simulink model "bomb"  (R2018b)
settings: Solver=FixedStepAuto  StartTime=0.0  StopTime=inf  FixedStep=0.01  RelTol=1e-3
values from neighbouring files (symbols this model uses):
  caliber = 0.299    [init.m]
  g = 9.8    [init.m]
  specified_drag_coefficient = 0.16    [init.m]
  standard_density = 1.225    [init.m]
  standard_drag_coefficient = 0.659    [init.m]
  standard_temperature = 288.4    [init.m]
  weight = 216.5    [init.m]
libraries: aerolibatmos2 x1, aerolibasang x1
settings Model: Creator=ysq  LastModifiedBy=ysq

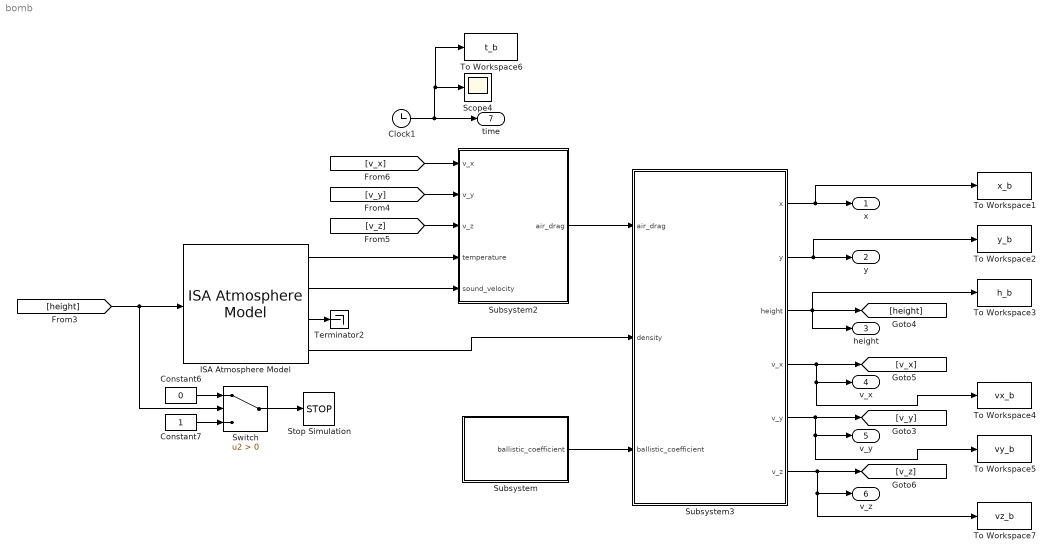
== system bomb ==
  Clock1 : Clock
  Constant6 : Constant  Value=0
  Constant7 : Constant
  ISA Atmosphere Model : aerolibatmos2/ISA Atmosphere Model  custom=off  g=9.80665  gamma=1.4  R=287.0531  L=0.0065  h_trop=11000  h_strat=20000  rho0=1.225  P0=101325  T0=288.15  h0=0
      settings: SourceProductName=Aerospace Blockset
  Scope4 : Scope
  Stop Simulation : Stop
  Subsystem : Subsystem
  Subsystem2 : Subsystem
  Subsystem3 : Subsystem
  Switch : Switch  Criteria=u2 > Threshold
  Terminator2 : Terminator
  To Workspace1 : ToWorkspace  VariableName=x_b  SampleTime=-1
  To Workspace2 : ToWorkspace  VariableName=y_b  SampleTime=-1
  To Workspace3 : ToWorkspace  VariableName=h_b  SampleTime=-1
  To Workspace4 : ToWorkspace  VariableName=vx_b  SampleTime=-1
  To Workspace5 : ToWorkspace  VariableName=vy_b  SampleTime=-1
  To Workspace6 : ToWorkspace  VariableName=t_b  SampleTime=-1
  To Workspace7 : ToWorkspace  VariableName=vz_b  SampleTime=-1
  x : Outport
  y : Outport  Port=2
  height : Outport  Port=3
  v_x : Outport  Port=4
  v_y : Outport  Port=5
  v_z : Outport  Port=6
  time : Outport  Port=7
  wires:
  Constant7/1 -> Switch/3
  [v_z] -> Subsystem2/3(v_z)
  [height] -> ISA Atmosphere Model/1, Switch/2
  Subsystem3/2(y) -> y/1, To Workspace2/1
  ISA Atmosphere Model/4 -> Subsystem3/2(density)
  Subsystem/1(ballistic_coefficient) -> Subsystem3/3(ballistic_coefficient)
  Subsystem3/3(height) -> height/1, To Workspace3/1, [height]
  ISA Atmosphere Model/1 -> Subsystem2/4(temperature)
  Subsystem3/4(v_x) -> To Workspace4/1, v_x/1, [v_x]
  Switch/1 -> Stop Simulation/1
  Subsystem2/1(air_drag) -> Subsystem3/1(air_drag)
  ISA Atmosphere Model/3 -> Terminator2/1
  Constant6/1 -> Switch/1
  Subsystem3/1(x) -> x/1, To Workspace1/1
  ISA Atmosphere Model/2 -> Subsystem2/5(sound_velocity)
  Clock1/1 -> time/1, To Workspace6/1, Scope4/1
  Subsystem3/5(v_y) -> To Workspace5/1, v_y/1, [v_y]
  [v_y] -> Subsystem2/2(v_y)
  [v_x] -> Subsystem2/1(v_x)
  Subsystem3/6(v_z) -> To Workspace7/1, v_z/1, [v_z]

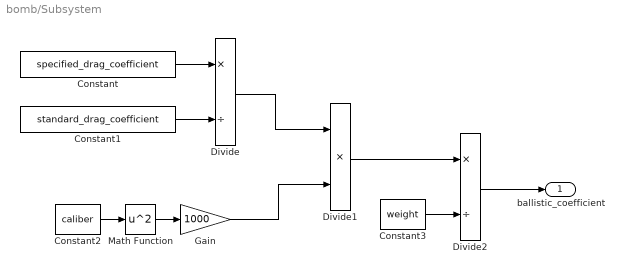
== system bomb/Subsystem ==
  Constant : Constant  Value=specified_drag_coefficient
  Constant1 : Constant  Value=standard_drag_coefficient
  Constant2 : Constant  Value=caliber
  Constant3 : Constant  Value=weight
  Divide : Product  Inputs=*/
  Divide1 : Product  Inputs=**
  Divide2 : Product  Inputs=*/
  Gain : Gain  Gain=1000
  Math Function : Math  Operator=square  SaturateOnIntegerOverflow=on
  ballistic_coefficient : Outport
  wires:
  Divide/1 -> Divide1/1
  Gain/1 -> Divide1/2
  Constant/1 -> Divide/1
  Math Function/1 -> Gain/1
  Constant3/1 -> Divide2/2
  Divide2/1 -> ballistic_coefficient/1
  Constant2/1 -> Math Function/1
  Constant1/1 -> Divide/2
  Divide1/1 -> Divide2/1

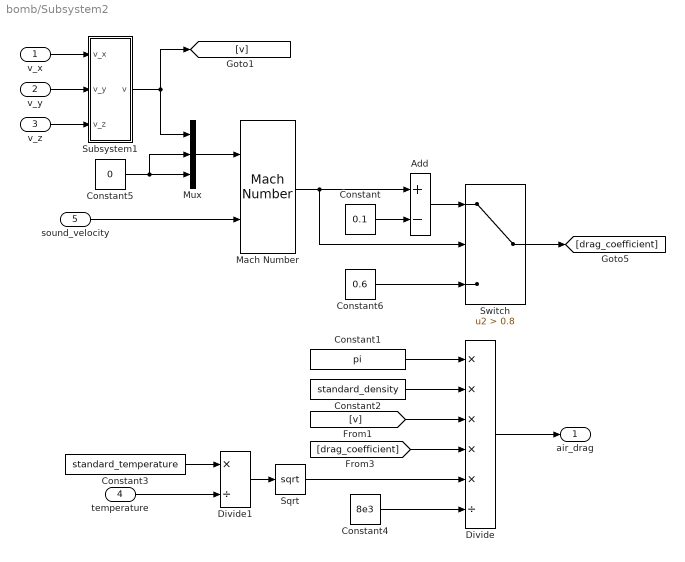
== system bomb/Subsystem2 ==
  v_x : Inport
  v_y : Inport  Port=2
  v_z : Inport  Port=3
  temperature : Inport  Port=4
  sound_velocity : Inport  Port=5
  Add : Sum  Inputs=+-
  Constant : Constant  Value=0.1
  Constant1 : Constant  Value=pi
  Constant2 : Constant  Value=standard_density
  Constant3 : Constant  Value=standard_temperature
  Constant4 : Constant  Value=8e3
  Constant5 : Constant  Value=0
  Constant6 : Constant  Value=0.6
  Divide : Product  Inputs=*****/
  Divide1 : Product  Inputs=*/
  Mach Number : aerolibasang/Mach Number
      settings: SourceProductName=Aerospace Blockset  SourceProductBaseCode=AE
  Mux : Mux  Inputs=3
  Sqrt : Sqrt  SaturateOnIntegerOverflow=on
  Subsystem1 : Subsystem
  Switch : Switch  Criteria=u2 > Threshold  Threshold=0.8
  air_drag : Outport
  wires:
  Switch/1 -> [drag_coefficient]
  [drag_coefficient] -> Divide/4
  Constant2/1 -> Divide/2
  v_x/1 -> Subsystem1/1(v_x)
  Divide1/1 -> Sqrt/1
  Constant1/1 -> Divide/1
  Mach Number/1 -> Switch/2, Add/1
  Sqrt/1 -> Divide/5
  Constant3/1 -> Divide1/1
  Constant4/1 -> Divide/6
  Constant/1 -> Add/2
  v_z/1 -> Subsystem1/3(v_z)
  Divide/1 -> air_drag/1
  Add/1 -> Switch/1
  [v] -> Divide/3
  temperature/1 -> Divide1/2
  sound_velocity/1 -> Mach Number/2
  Mux/1 -> Mach Number/1
  Constant5/1 -> Mux/2, Mux/3
  Subsystem1/1(v) -> Mux/1, [v]
  v_y/1 -> Subsystem1/2(v_y)
  Constant6/1 -> Switch/3

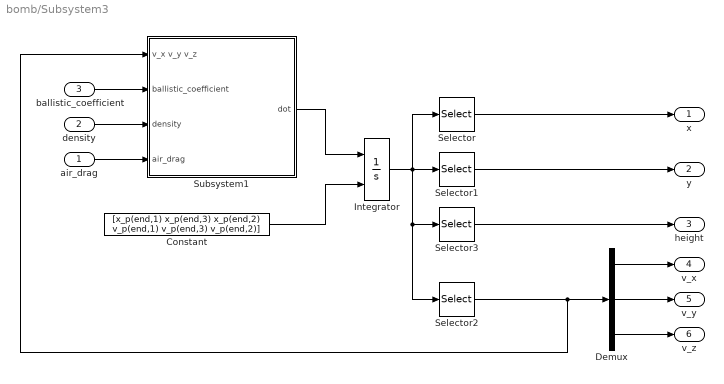
== system bomb/Subsystem3 ==
  air_drag : Inport
  density : Inport  Port=2
  ballistic_coefficient : Inport  Port=3
  Constant : Constant  Value=[x_p(end,1) x_p(end,3) x_p(end,2) v_p(end,1) v_p(end,3) v_p(end,2)]
  Demux : Demux  Outputs=3
  Integrator : Integrator  InitialConditionSource=external
  Selector : Selector  InputPortWidth=6  IndexOptions=Index vector (dialog)  Indices=[1]  OutputSizes=1
  Selector1 : Selector  InputPortWidth=6  IndexOptions=Index vector (dialog)  Indices=[2]  OutputSizes=1
  Selector2 : Selector  InputPortWidth=6  IndexOptions=Index vector (dialog)  Indices=[4 5 6]  OutputSizes=1
  Selector3 : Selector  InputPortWidth=6  IndexOptions=Index vector (dialog)  Indices=[3]  OutputSizes=1
  Subsystem1 : Subsystem
  x : Outport
  y : Outport  Port=2
  height : Outport  Port=3
  v_x : Outport  Port=4
  v_y : Outport  Port=5
  v_z : Outport  Port=6
  wires:
  Integrator/1 -> Selector2/1, Selector3/1, Selector/1, Selector1/1
  Constant/1 -> Integrator/2
  ballistic_coefficient/1 -> Subsystem1/2(ballistic_coefficient)
  air_drag/1 -> Subsystem1/4(air_drag)
  Demux/3 -> v_z/1
  density/1 -> Subsystem1/3(density)
  Selector2/1 -> Demux/1, Subsystem1/1(v_x v_y v_z)
  Subsystem1/1(dot) -> Integrator/1
  Demux/1 -> v_x/1
  Selector3/1 -> height/1
  Demux/2 -> v_y/1
  Selector1/1 -> y/1
  Selector/1 -> x/1

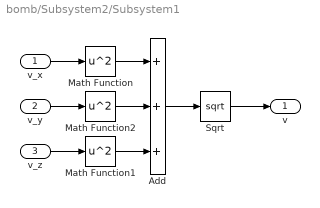
== system bomb/Subsystem2/Subsystem1 ==
  v_x : Inport
  v_y : Inport  Port=2
  v_z : Inport  Port=3
  Add : Sum  Inputs=+++
  Math Function : Math  Operator=square  SaturateOnIntegerOverflow=on
  Math Function1 : Math  Operator=square  SaturateOnIntegerOverflow=on
  Math Function2 : Math  Operator=square  SaturateOnIntegerOverflow=on
  Sqrt : Sqrt  SaturateOnIntegerOverflow=on
  v : Outport
  wires:
  Add/1 -> Sqrt/1
  v_x/1 -> Math Function/1
  Sqrt/1 -> v/1
  Math Function/1 -> Add/1
  v_z/1 -> Math Function1/1
  Math Function1/1 -> Add/3
  Math Function2/1 -> Add/2
  v_y/1 -> Math Function2/1

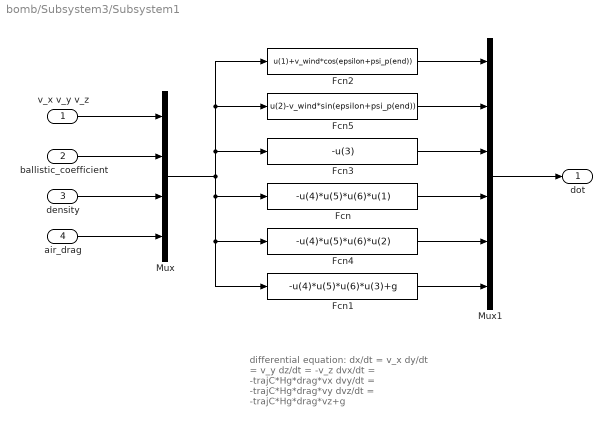
== system bomb/Subsystem3/Subsystem1 ==
  note: differential equation:
      | dx/dt = v_x
      | dy/dt = v_y
      | dz/dt = -v_z
      | dvx/dt = -trajC*Hg*drag*vx
      | dvy/dt = -trajC*Hg*drag*vy
      | dvz/dt = -trajC*Hg*drag*vz+g
  v_x v_y v_z : Inport
  ballistic_coefficient : Inport  Port=2
  density : Inport  Port=3
  air_drag : Inport  Port=4
  Fcn : Fcn  Expr=-u(4)*u(5)*u(6)*u(1)
  Fcn1 : Fcn  Expr=-u(4)*u(5)*u(6)*u(3)+g
  Fcn2 : Fcn  Expr=u(1)+v_wind*cos(epsilon+psi_p(end))
  Fcn3 : Fcn  Expr=-u(3)
  Fcn4 : Fcn  Expr=-u(4)*u(5)*u(6)*u(2)
  Fcn5 : Fcn  Expr=u(2)-v_wind*sin(epsilon+psi_p(end))
  Mux : Mux
  Mux1 : Mux  Inputs=6
  dot : Outport
  wires:
  Mux/1 -> Fcn5/1, Fcn2/1, Fcn3/1, Fcn4/1, Fcn1/1, Fcn/1
  Mux1/1 -> dot/1
  Fcn3/1 -> Mux1/3
  Fcn2/1 -> Mux1/1
  v_x v_y v_z/1 -> Mux/1
  Fcn1/1 -> Mux1/6
  Fcn/1 -> Mux1/4
  ballistic_coefficient/1 -> Mux/2
  density/1 -> Mux/3
  air_drag/1 -> Mux/4
  Fcn4/1 -> Mux1/5
  Fcn5/1 -> Mux1/2
